simulink model "Pendulo_Adaptativo"  (R2023b)
settings: Solver=ode45  StartTime=0.0  StopTime=82  MaxStep=0.02  RelTol=1e-3
model workspace (MAT data in the model file):
  longitud = Simulink.Parameter
  longitud.Value = 0.6
  longitud.DataType = 'auto'
  longitud.Complexity = 'real'
  longitud.Dimensions = [1 1]
libraries: slpidlib x5
settings Model: Creator=Usuario  LastModifiedBy=Usuario
settings SolverCC: DaesscMode=Fast  ZeroCrossAlgorithm=Adaptive  EnableFixedStepZeroCrossing=on
settings DebuggingCC: IgnoredZcDiagnostic=none

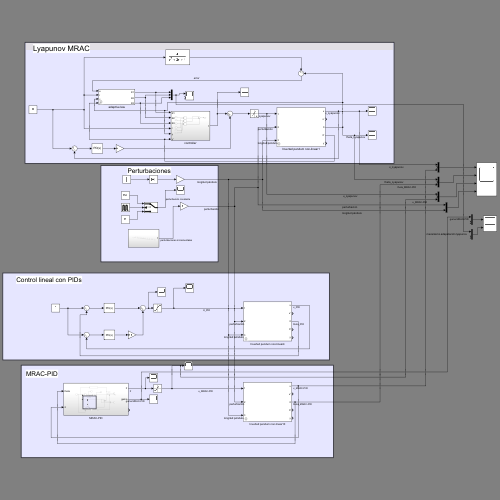
[thumbnail: Simulink's stored preview of the top-level diagram]
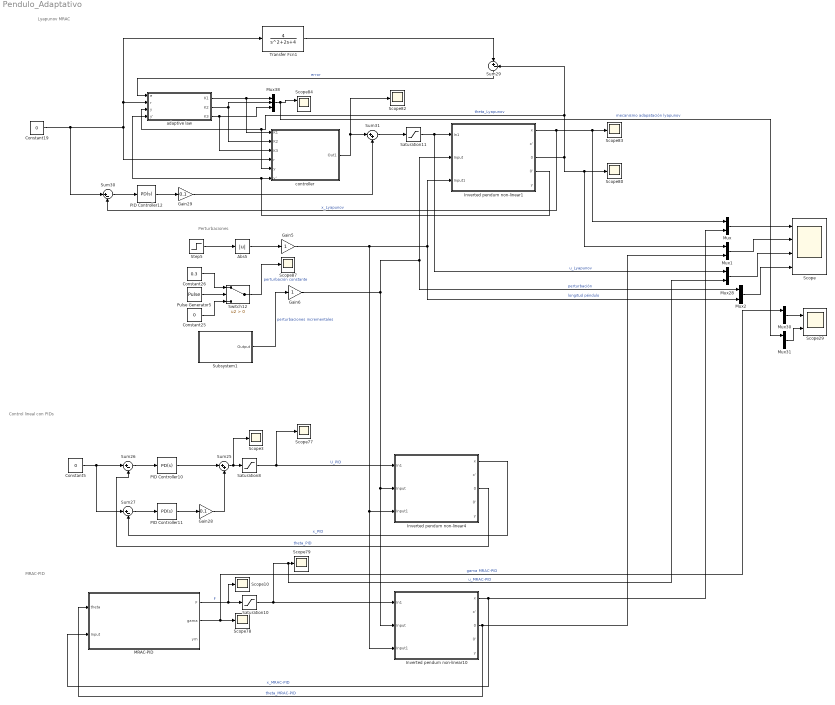
== system Pendulo_Adaptativo ==
  note: Lyapunov MRAC
  note: Perturbaciones
  note: Control lineal con PIDs
  note: MRAC-PID
  Abs5 : Abs  SaturateOnIntegerOverflow=off
  Constant19 : Constant  Value=0
  Constant25 : Constant  Value=0
  Constant26 : Constant  Value=0.3
  Constant5 : Constant  Value=0
  Gain28 : Gain  Gain=0.1
  Gain29 : Gain  Gain=0.1
  Gain5 : Gain
  Gain6 : Gain
  Inverted pendum non-linear1 : Subsystem  mask{M_=2, L=0.6, g=9.8, angulo=0.2, m=0.2}
      mask prompts: M_ "M"; angulo "angulo inicial"
  Inverted pendum non-linear10 : Subsystem  mask{M_=2, L=0.6, g=9.8, angulo=0.2, m=0.2}
      mask prompts: M_ "M"; angulo "angulo inicial"
  Inverted pendum non-linear4 : Subsystem  mask{M_=2, L=0.6, g=9.8, angulo=0.2, m=0.2}
      mask prompts: M_ "M"; angulo "angulo inicial"
  MRAC-PID : Subsystem
  Mux{,1,28,38} (4 alike) : Mux  Inputs=3
  Mux2 : Mux  Inputs=2
  Mux30 : Mux  Inputs=2
  Mux31 : Mux  Inputs=2
  PID Controller10 : slpidlib/PID Controller  Controller=PD  Form=Parallel  TimeDomain=Continuous-time  UseExternalTs=off  SampleTime=-1  IntegratorMethod=Forward Euler  FilterMethod=Forward Euler  ControllerParametersSource=internal  P=-30  I=0.01  UseKiTs=off  D=-10  N=100  UseFilter=on  TunerSelectOption=Transfer Function Based (PID Tuner App)  InitialConditionSource=internal  InitialConditionForIntegrator=0  InitialConditionForFilter=0  DifferentiatorICPrevScaledInput=0  ExternalReset=none  TrackingMode=off  Kt=1  LimitOutput=off  SatLimitsSource=internal  UpperSaturationLimit=inf  LowerSaturationLimit=-inf  LinearizeAsGain=on  AntiWindupMode=none  Kb=1  LimitIntegrator=off  UpperIntegratorSaturationLimit=inf  LowerIntegratorSaturationLimit=-inf  POutMin=[]  POutMax=[]  IOutMin=[]  IOutMax=[]  DOutMin=[]  DOutMax=[]  NOutMin=[]  NOutMax=[]  SumOutMin=[]  SumOutMax=[]  SaturationOutMin=[]  SaturationOutMax=[]  PParamMin=[]  PParamMax=[]  IParamMin=[]  IParamMax=[]  DParamMin=[]  DParamMax=[]  NParamMin=[]  NParamMax=[]  KbParamMin=[]  KbParamMax=[]  KtParamMin=[]  KtParamMax=[]  KbOutMin=[]  KbOutMax=[]  KtOutMin=[]  KtOutMax=[]  IntegratorOutMin=[]  IntegratorOutMax=[]  FilterOutMin=[]  FilterOutMax=[]  SumI1OutMin=[]  SumI1OutMax=[]  SumI2OutMin=[]  SumI2OutMax=[]  SumI3OutMin=[]  SumI3OutMax=[]  SumI4OutMin=[]  SumI4OutMax=[]  SumDOutMin=[]  SumDOutMax=[]  DifferentiatorOutMin=[]  DifferentiatorOutMax=[]  FilterDiffOutCoefMin=[]  FilterDiffOutCoefMax=[]  ReciprocalOutMin=[]  ReciprocalOutMax=[]  SumDenOutMin=[]  SumDenOutMax=[]  SumNumOutMin=[]  SumNumOutMax=[]  DivideOutMin=[]  DivideOutMax=[]  UdiffTsProdOutMin=[]  UdiffTsProdOutMax=[]  NTsProdOutMin=[]  NTsProdOutMax=[]  UintegralTsProdOutMin=[]  UintegralTsProdOutMax=[]  UngainTsProdOutMin=[]  UngainTsProdOutMax=[]  ClampingZeroOutDataTypeStr=Inherit: Inherit via back propagation  ClampingZeroOutMin=[]  ClampingZeroOutMax=[]  FilterDenConstantOutDataTypeStr=Inherit: Inherit via back propagation  FilterDenConstantOutMin=[]  FilterDenConstantOutMax=[]  PCopyOutDataTypeStr=Inherit: Inherit via back propagation  PCopyOutMin=[]  PCopyOutMax=[]  NCopyOutDataTypeStr=Inherit: Inherit via back propagation  NCopyOutMin=[]  NCopyOutMax=[]  IntegratorContinuousStateAttributes=''  IntegratorStateMustResolveToSignalObject=off  IntegratorRTWStateStorageClass=Auto  FilterContinuousStateAttributes=''  FilterStateMustResolveToSignalObject=off  FilterRTWStateStorageClass=Auto  ParallelPVariant=InternalParameters  IdealPVariant=Disabled  IVariant=Disabled  DVariant=InternalParameters  IntegratorVariant=Disabled  SatVariant=Disabled  AWVariant=Disabled  PCopyVariant=Disabled  TRVariant=Disabled  FdbkBlocksVariant=Forward  IdealPFdbkVariant=Disabled  SatFdbkVariant=Disabled  DerivativeFilterVariant=ContFilter  NVariant=InternalParameters  NCopyVariant=Disabled  FilterICVariant=InternalICsFilter  IntegratorICVariant=Disabled  ExternalResetVariant=Disabled  TRSumVariant=Passthrough  SumFdbkVariant=Disabled  SumVariant=Sum_PD  TsampFilterVariant=InternalTs  TsampNgainVariant=Passthrough  TsampIntegralVariant=Disabled_SignalSpec  ExternalSaturationOutDataTypeStr=Inherit: Same as second input
  PID Controller11 : slpidlib/PID Controller  Controller=PD  Form=Parallel  TimeDomain=Continuous-time  UseExternalTs=off  SampleTime=-1  IntegratorMethod=Forward Euler  FilterMethod=Forward Euler  ControllerParametersSource=internal  P=-3.5  I=0.01  UseKiTs=off  D=-10  N=10  UseFilter=on  TunerSelectOption=Transfer Function Based (PID Tuner App)  InitialConditionSource=internal  InitialConditionForIntegrator=0  InitialConditionForFilter=0  DifferentiatorICPrevScaledInput=0  ExternalReset=none  TrackingMode=off  Kt=1  LimitOutput=off  SatLimitsSource=internal  UpperSaturationLimit=inf  LowerSaturationLimit=-inf  LinearizeAsGain=on  AntiWindupMode=none  Kb=1  LimitIntegrator=off  UpperIntegratorSaturationLimit=inf  LowerIntegratorSaturationLimit=-inf  POutMin=[]  POutMax=[]  IOutMin=[]  IOutMax=[]  DOutMin=[]  DOutMax=[]  NOutMin=[]  NOutMax=[]  SumOutMin=[]  SumOutMax=[]  SaturationOutMin=[]  SaturationOutMax=[]  PParamMin=[]  PParamMax=[]  IParamMin=[]  IParamMax=[]  DParamMin=[]  DParamMax=[]  NParamMin=[]  NParamMax=[]  KbParamMin=[]  KbParamMax=[]  KtParamMin=[]  KtParamMax=[]  KbOutMin=[]  KbOutMax=[]  KtOutMin=[]  KtOutMax=[]  IntegratorOutMin=[]  IntegratorOutMax=[]  FilterOutMin=[]  FilterOutMax=[]  SumI1OutMin=[]  SumI1OutMax=[]  SumI2OutMin=[]  SumI2OutMax=[]  SumI3OutMin=[]  SumI3OutMax=[]  SumI4OutMin=[]  SumI4OutMax=[]  SumDOutMin=[]  SumDOutMax=[]  DifferentiatorOutMin=[]  DifferentiatorOutMax=[]  FilterDiffOutCoefMin=[]  FilterDiffOutCoefMax=[]  ReciprocalOutMin=[]  ReciprocalOutMax=[]  SumDenOutMin=[]  SumDenOutMax=[]  SumNumOutMin=[]  SumNumOutMax=[]  DivideOutMin=[]  DivideOutMax=[]  UdiffTsProdOutMin=[]  UdiffTsProdOutMax=[]  NTsProdOutMin=[]  NTsProdOutMax=[]  UintegralTsProdOutMin=[]  UintegralTsProdOutMax=[]  UngainTsProdOutMin=[]  UngainTsProdOutMax=[]  ClampingZeroOutDataTypeStr=Inherit: Inherit via back propagation  ClampingZeroOutMin=[]  ClampingZeroOutMax=[]  FilterDenConstantOutDataTypeStr=Inherit: Inherit via back propagation  FilterDenConstantOutMin=[]  FilterDenConstantOutMax=[]  PCopyOutDataTypeStr=Inherit: Inherit via back propagation  PCopyOutMin=[]  PCopyOutMax=[]  NCopyOutDataTypeStr=Inherit: Inherit via back propagation  NCopyOutMin=[]  NCopyOutMax=[]  IntegratorContinuousStateAttributes=''  IntegratorStateMustResolveToSignalObject=off  IntegratorRTWStateStorageClass=Auto  FilterContinuousStateAttributes=''  FilterStateMustResolveToSignalObject=off  FilterRTWStateStorageClass=Auto  ParallelPVariant=InternalParameters  IdealPVariant=Disabled  IVariant=Disabled  DVariant=InternalParameters  IntegratorVariant=Disabled  SatVariant=Disabled  AWVariant=Disabled  PCopyVariant=Disabled  TRVariant=Disabled  FdbkBlocksVariant=Forward  IdealPFdbkVariant=Disabled  SatFdbkVariant=Disabled  DerivativeFilterVariant=ContFilter  NVariant=InternalParameters  NCopyVariant=Disabled  FilterICVariant=InternalICsFilter  IntegratorICVariant=Disabled  ExternalResetVariant=Disabled  TRSumVariant=Passthrough  SumFdbkVariant=Disabled  SumVariant=Sum_PD  TsampFilterVariant=InternalTs  TsampNgainVariant=Passthrough  TsampIntegralVariant=Disabled_SignalSpec  ExternalSaturationOutDataTypeStr=Inherit: Same as second input
  PID Controller12 : slpidlib/PID Controller  Controller=PD  Form=Parallel  TimeDomain=Continuous-time  UseExternalTs=off  SampleTime=-1  IntegratorMethod=Forward Euler  FilterMethod=Forward Euler  ControllerParametersSource=internal  P=-3.5  I=0.01  UseKiTs=off  D=-10  N=10  UseFilter=on  TunerSelectOption=Transfer Function Based (PID Tuner App)  InitialConditionSource=internal  InitialConditionForIntegrator=0  InitialConditionForFilter=0  DifferentiatorICPrevScaledInput=0  ExternalReset=none  TrackingMode=off  Kt=1  LimitOutput=off  SatLimitsSource=internal  UpperSaturationLimit=inf  LowerSaturationLimit=-inf  LinearizeAsGain=on  AntiWindupMode=none  Kb=1  LimitIntegrator=off  UpperIntegratorSaturationLimit=inf  LowerIntegratorSaturationLimit=-inf  POutMin=[]  POutMax=[]  IOutMin=[]  IOutMax=[]  DOutMin=[]  DOutMax=[]  NOutMin=[]  NOutMax=[]  SumOutMin=[]  SumOutMax=[]  SaturationOutMin=[]  SaturationOutMax=[]  PParamMin=[]  PParamMax=[]  IParamMin=[]  IParamMax=[]  DParamMin=[]  DParamMax=[]  NParamMin=[]  NParamMax=[]  KbParamMin=[]  KbParamMax=[]  KtParamMin=[]  KtParamMax=[]  KbOutMin=[]  KbOutMax=[]  KtOutMin=[]  KtOutMax=[]  IntegratorOutMin=[]  IntegratorOutMax=[]  FilterOutMin=[]  FilterOutMax=[]  SumI1OutMin=[]  SumI1OutMax=[]  SumI2OutMin=[]  SumI2OutMax=[]  SumI3OutMin=[]  SumI3OutMax=[]  SumI4OutMin=[]  SumI4OutMax=[]  SumDOutMin=[]  SumDOutMax=[]  DifferentiatorOutMin=[]  DifferentiatorOutMax=[]  FilterDiffOutCoefMin=[]  FilterDiffOutCoefMax=[]  ReciprocalOutMin=[]  ReciprocalOutMax=[]  SumDenOutMin=[]  SumDenOutMax=[]  SumNumOutMin=[]  SumNumOutMax=[]  DivideOutMin=[]  DivideOutMax=[]  UdiffTsProdOutMin=[]  UdiffTsProdOutMax=[]  NTsProdOutMin=[]  NTsProdOutMax=[]  UintegralTsProdOutMin=[]  UintegralTsProdOutMax=[]  UngainTsProdOutMin=[]  UngainTsProdOutMax=[]  ClampingZeroOutDataTypeStr=Inherit: Inherit via back propagation  ClampingZeroOutMin=[]  ClampingZeroOutMax=[]  FilterDenConstantOutDataTypeStr=Inherit: Inherit via back propagation  FilterDenConstantOutMin=[]  FilterDenConstantOutMax=[]  PCopyOutDataTypeStr=Inherit: Inherit via back propagation  PCopyOutMin=[]  PCopyOutMax=[]  NCopyOutDataTypeStr=Inherit: Inherit via back propagation  NCopyOutMin=[]  NCopyOutMax=[]  IntegratorContinuousStateAttributes=''  IntegratorStateMustResolveToSignalObject=off  IntegratorRTWStateStorageClass=Auto  FilterContinuousStateAttributes=''  FilterStateMustResolveToSignalObject=off  FilterRTWStateStorageClass=Auto  ParallelPVariant=InternalParameters  IdealPVariant=Disabled  IVariant=Disabled  DVariant=InternalParameters  IntegratorVariant=Disabled  SatVariant=Disabled  AWVariant=Disabled  PCopyVariant=Disabled  TRVariant=Disabled  FdbkBlocksVariant=Forward  IdealPFdbkVariant=Disabled  SatFdbkVariant=Disabled  DerivativeFilterVariant=ContFilter  NVariant=InternalParameters  NCopyVariant=Disabled  FilterICVariant=InternalICsFilter  IntegratorICVariant=Disabled  ExternalResetVariant=Disabled  TRSumVariant=Passthrough  SumFdbkVariant=Disabled  SumVariant=Sum_PD  TsampFilterVariant=InternalTs  TsampNgainVariant=Passthrough  TsampIntegralVariant=Disabled_SignalSpec  ExternalSaturationOutDataTypeStr=Inherit: Same as second input
  Pulse Generator5 : DiscretePulseGenerator  PulseType=Time based  Period=10  PhaseDelay=10
  Saturation10 : Saturate  UpperLimit=10  LowerLimit=-10
  Saturation11 : Saturate  UpperLimit=10  LowerLimit=-10
  Saturation8 : Saturate  UpperLimit=10  LowerLimit=-10
  Scope : Scope  NumInputPorts=4
  Scope{3,10,77..80,82..83,87} (9 alike) : Scope
  Scope29 : Scope  NumInputPorts=2
  Scope84 : Scope  NumInputPorts=2
  Step5 : Step  Time=30.5  Before=0.6  After=2  SampleTime=0
  Subsystem1 : Subsystem
  Sum25 : Sum  Inputs=|++
  Sum{26..27,29..30} (4 alike) : Sum  Inputs=|+-
  Sum31 : Sum  Inputs=|++
  Switch12 : Switch  Criteria=u2 > Threshold  SaturateOnIntegerOverflow=off  InputSameDT=off
  Transfer Fcn1 : TransferFcn  Numerator=[4]  Denominator=[1 2 4]
  adaptive law : Subsystem  mask{p12=1/8, p22=5/16, gama1=-100, gama2=100, gama3=100, k1=-10, k2=-40, k3=-10}
  controller : Subsystem
  wires:
  PID Controller10/1 -> Sum25/1
  PID Controller11/1 -> Gain28/1
  Gain28/1 -> Sum25/2
  Sum26/1 -> PID Controller10/1
  Constant5/1 -> Sum27/1, Sum26/1
  Inverted pendum non-linear4/3(0) -> Sum26/2  "theta_PID"
  Inverted pendum non-linear4/1(x) -> Sum27/2  "x_PID"
  Sum27/1 -> PID Controller11/1
  Mux1/1 -> Scope/2
  Mux/1 -> Scope/1
  Mux28/1 -> Scope/3
  Sum25/1 -> Scope3/1, Saturation8/1
  Saturation8/1 -> Scope77/1, Inverted pendum non-linear4/1(In1)  "U_PID"
  Saturation10/1 -> Mux28/3, Scope79/1, Inverted pendum non-linear10/1(In1)  "u_MRAC-PID"
  MRAC-PID/1(F) -> Scope10/1, Saturation10/1  "F"
  MRAC-PID/2(gama) -> Mux30/1, Scope78/1  "gama MRAC-PID"
  Inverted pendum non-linear10/1(x) -> Mux/3, MRAC-PID/2(Input)  "x_MRAC-PID"
  Inverted pendum non-linear10/3(0) -> Mux1/3, MRAC-PID/1(theta)  "theta_MRAC-PID"
  adaptive law/2(K2) -> Mux38/2, controller/2(K2)
  adaptive law/3(K3) -> controller/3(K3), Mux38/3
  Constant19/1 -> controller/4(r), Transfer Fcn1/1, adaptive law/2(r), Sum30/1
  controller/1(Out1) -> Sum31/1, Scope82/1
  Transfer Fcn1/1 -> Sum29/1
  Inverted pendum non-linear1/3(0) -> Sum29/2, adaptive law/3(y), controller/5(y), Mux1/1, Scope80/1  "theta_Lyapunov"
  Sum29/1 -> adaptive law/1(e)  "error"
  Inverted pendum non-linear1/4(0') -> adaptive law/4(y'), controller/6(y')
  Inverted pendum non-linear1/1(x) -> Mux/1, Scope83/1, Sum30/2  "x_Lyapunov"
  adaptive law/1(K1) -> Mux38/1, controller/1(K1)
  Mux38/1 -> Mux31/1, Scope84/1  "mecanismo adapatación lyapunov"
  Switch12/1 -> Scope87/1  "perturbación constante"
  Constant26/1 -> Switch12/1
  Constant25/1 -> Switch12/3
  Pulse Generator5/1 -> Switch12/2
  Step5/1 -> Abs5/1
  PID Controller12/1 -> Gain29/1
  Sum30/1 -> PID Controller12/1
  Sum31/1 -> Saturation11/1
  Gain29/1 -> Sum31/2
  Saturation11/1 -> Mux28/1, Inverted pendum non-linear1/1(In1)  "u_Lyapunov"
  Mux2/1 -> Scope/4
  Gain5/1 -> Inverted pendum non-linear4/3(Input1), Inverted pendum non-linear10/3(Input1), Mux2/2, Inverted pendum non-linear1/3(Input1)  "longitud péndulo"
  Gain6/1 -> Mux2/1, Inverted pendum non-linear1/2(Input), Inverted pendum non-linear4/2(Input), Inverted pendum non-linear10/2(Input)  "perturbación"
  Abs5/1 -> Gain5/1
  Mux30/1 -> Scope29/1
  Mux31/1 -> Scope29/2
  Subsystem1/1(Output) -> Gain6/1  "perturbaciones incrementales"

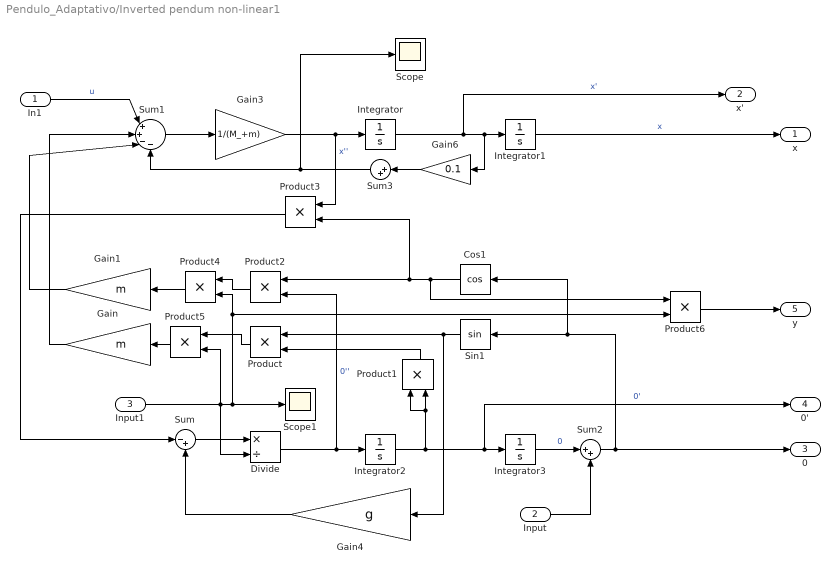
== system Pendulo_Adaptativo/Inverted pendum non-linear1 ==
  In1 : Inport
  Input : Inport  Port=2
  Input1 : Inport  Port=3
  Cos1 : Trigonometry  Operator=cos
  Divide : Product  Inputs=*/
  Gain : Gain  Gain=m
  Gain1 : Gain  Gain=m
  Gain3 : Gain  Gain=1/(M_+m)
  Gain4 : Gain  Gain=g
  Gain6 : Gain  Gain=0.1
  Integrator : Integrator
  Integrator1 : Integrator
  Integrator2 : Integrator
  Integrator3 : Integrator  InitialCondition=angulo
  Product{,1..6} (7 alike) : Product
  Scope : Scope
  Scope1 : Scope
  Sin1 : Trigonometry
  Sum : Sum  Inputs=|-+
  Sum1 : Sum  Inputs=|++--
  Sum2 : Sum  Inputs=|++
  Sum3 : Sum  Inputs=|++
  x : Outport
  x' : Outport  Port=2
  0 : Outport  Port=3
  0' : Outport  Port=4
  y : Outport  Port=5
  wires:
  Integrator2/1 -> Product1/1, Product1/2, Integrator3/1, 0'/1  "0'"
  Integrator1/1 -> x/1  "x"
  Integrator3/1 -> Sum2/1  "0"
  Cos1/1 -> Product6/1, Product3/2, Product2/1
  Sin1/1 -> Gain4/1, Product/1
  Product1/1 -> Product/2
  Gain/1 -> Sum1/2
  Gain1/1 -> Sum1/3
  Product3/1 -> Sum/1
  Gain4/1 -> Sum/2
  Sum1/1 -> Gain3/1
  Gain3/1 -> Product3/1, Integrator/1  "x''"
  In1/1 -> Sum1/1  "u"
  Sum/1 -> Divide/1
  Divide/1 -> Product2/2, Integrator2/1  "0''"
  Product6/1 -> y/1
  Sum2/1 -> Cos1/1, Sin1/1, 0/1
  Input/1 -> Sum2/2
  Product4/1 -> Gain1/1
  Product2/1 -> Product4/1
  Input1/1 -> Product5/2, Scope1/1, Product6/2, Product4/2, Divide/2
  Product5/1 -> Gain/1
  Product/1 -> Product5/1
  Sum3/1 -> Scope/1, Sum1/4
  Gain6/1 -> Sum3/1
  Integrator/1 -> Gain6/1, Integrator1/1, x'/1  "x'"

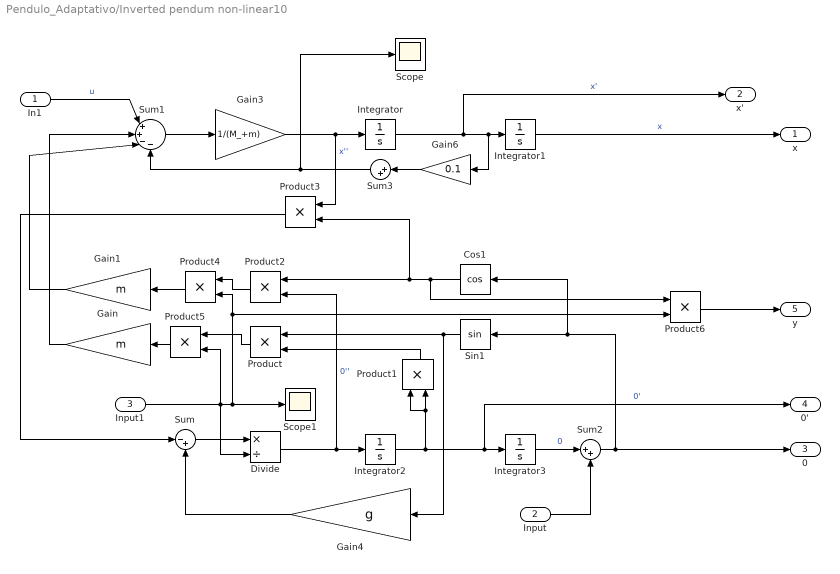
== system Pendulo_Adaptativo/Inverted pendum non-linear10 ==
  In1 : Inport
  Input : Inport  Port=2
  Input1 : Inport  Port=3
  Cos1 : Trigonometry  Operator=cos
  Divide : Product  Inputs=*/
  Gain : Gain  Gain=m
  Gain1 : Gain  Gain=m
  Gain3 : Gain  Gain=1/(M_+m)
  Gain4 : Gain  Gain=g
  Gain6 : Gain  Gain=0.1
  Integrator : Integrator
  Integrator1 : Integrator
  Integrator2 : Integrator
  Integrator3 : Integrator  InitialCondition=angulo
  Product{,1..6} (7 alike) : Product
  Scope : Scope
  Scope1 : Scope
  Sin1 : Trigonometry
  Sum : Sum  Inputs=|-+
  Sum1 : Sum  Inputs=|++--
  Sum2 : Sum  Inputs=|++
  Sum3 : Sum  Inputs=|++
  x : Outport
  x' : Outport  Port=2
  0 : Outport  Port=3
  0' : Outport  Port=4
  y : Outport  Port=5
  wires:
  Integrator/1 -> Gain6/1, Integrator1/1, x'/1  "x'"
  Integrator2/1 -> Product1/1, Product1/2, Integrator3/1, 0'/1  "0'"
  Integrator1/1 -> x/1  "x"
  Integrator3/1 -> Sum2/1  "0"
  Cos1/1 -> Product6/1, Product3/2, Product2/1
  Sin1/1 -> Gain4/1, Product/1
  Product1/1 -> Product/2
  Gain/1 -> Sum1/2
  Gain1/1 -> Sum1/3
  Product3/1 -> Sum/1
  Gain4/1 -> Sum/2
  Sum1/1 -> Gain3/1
  Gain3/1 -> Product3/1, Integrator/1  "x''"
  In1/1 -> Sum1/1  "u"
  Sum/1 -> Divide/1
  Divide/1 -> Product2/2, Integrator2/1  "0''"
  Product6/1 -> y/1
  Sum2/1 -> Cos1/1, Sin1/1, 0/1
  Input/1 -> Sum2/2
  Product4/1 -> Gain1/1
  Product2/1 -> Product4/1
  Input1/1 -> Product5/2, Scope1/1, Product6/2, Product4/2, Divide/2
  Product5/1 -> Gain/1
  Product/1 -> Product5/1
  Sum3/1 -> Scope/1, Sum1/4
  Gain6/1 -> Sum3/1

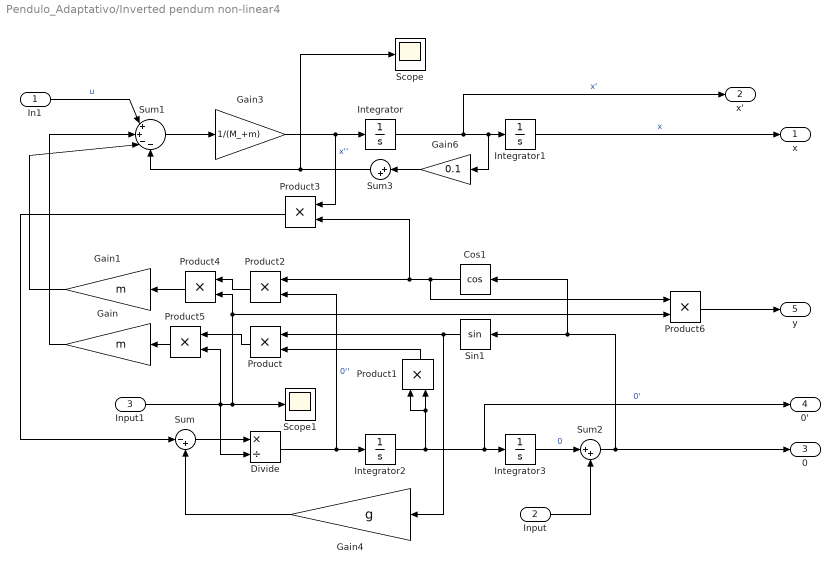
== system Pendulo_Adaptativo/Inverted pendum non-linear4 ==
  In1 : Inport
  Input : Inport  Port=2
  Input1 : Inport  Port=3
  Cos1 : Trigonometry  Operator=cos
  Divide : Product  Inputs=*/
  Gain : Gain  Gain=m
  Gain1 : Gain  Gain=m
  Gain3 : Gain  Gain=1/(M_+m)
  Gain4 : Gain  Gain=g
  Gain6 : Gain  Gain=0.1
  Integrator : Integrator
  Integrator1 : Integrator
  Integrator2 : Integrator
  Integrator3 : Integrator  InitialCondition=angulo
  Product{,1..6} (7 alike) : Product
  Scope : Scope
  Scope1 : Scope
  Sin1 : Trigonometry
  Sum : Sum  Inputs=|-+
  Sum1 : Sum  Inputs=|++--
  Sum2 : Sum  Inputs=|++
  Sum3 : Sum  Inputs=|++
  x : Outport
  x' : Outport  Port=2
  0 : Outport  Port=3
  0' : Outport  Port=4
  y : Outport  Port=5
  wires:
  Integrator2/1 -> Product1/1, Product1/2, Integrator3/1, 0'/1  "0'"
  Integrator1/1 -> x/1  "x"
  Integrator3/1 -> Sum2/1  "0"
  Cos1/1 -> Product6/1, Product3/2, Product2/1
  Sin1/1 -> Gain4/1, Product/1
  Product1/1 -> Product/2
  Gain/1 -> Sum1/2
  Gain1/1 -> Sum1/3
  Product3/1 -> Sum/1
  Gain4/1 -> Sum/2
  Sum1/1 -> Gain3/1
  Gain3/1 -> Product3/1, Integrator/1  "x''"
  In1/1 -> Sum1/1  "u"
  Sum/1 -> Divide/1
  Divide/1 -> Product2/2, Integrator2/1  "0''"
  Product6/1 -> y/1
  Sum2/1 -> Cos1/1, Sin1/1, 0/1
  Input/1 -> Sum2/2
  Product4/1 -> Gain1/1
  Product2/1 -> Product4/1
  Input1/1 -> Product5/2, Scope1/1, Product6/2, Product4/2, Divide/2
  Product5/1 -> Gain/1
  Product/1 -> Product5/1
  Sum3/1 -> Scope/1, Sum1/4
  Gain6/1 -> Sum3/1
  Integrator/1 -> Gain6/1, Integrator1/1, x'/1  "x'"

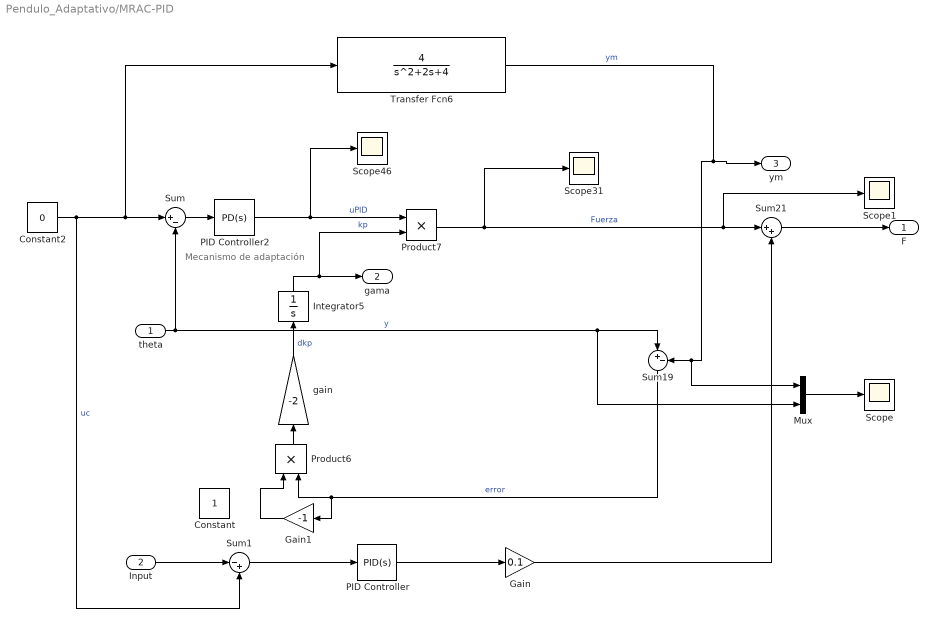
== system Pendulo_Adaptativo/MRAC-PID ==
  note: Mecanismo de adaptación
  theta : Inport
  Input : Inport  Port=2
  Constant : Constant
  Constant2 : Constant  Value=0
  Gain : Gain  Gain=0.1
  Gain1 : Gain  Gain=-1
  Integrator5 : Integrator  InitialCondition=2
  Mux : Mux  Inputs=2
  PID Controller : slpidlib/PID Controller  Controller=PID  Form=Parallel  TimeDomain=Continuous-time  UseExternalTs=off  SampleTime=-1  IntegratorMethod=Forward Euler  FilterMethod=Forward Euler  ControllerParametersSource=internal  P=-3.5  I=0  UseKiTs=off  D=-10  N=10  UseFilter=on  TunerSelectOption=Transfer Function Based (PID Tuner App)  InitialConditionSource=internal  InitialConditionForIntegrator=0  InitialConditionForFilter=0  DifferentiatorICPrevScaledInput=0  ExternalReset=none  TrackingMode=off  Kt=1  LimitOutput=off  SatLimitsSource=internal  UpperSaturationLimit=inf  LowerSaturationLimit=-inf  LinearizeAsGain=on  AntiWindupMode=none  Kb=1  LimitIntegrator=off  UpperIntegratorSaturationLimit=inf  LowerIntegratorSaturationLimit=-inf  POutMin=[]  POutMax=[]  IOutMin=[]  IOutMax=[]  DOutMin=[]  DOutMax=[]  NOutMin=[]  NOutMax=[]  SumOutMin=[]  SumOutMax=[]  SaturationOutMin=[]  SaturationOutMax=[]  PParamMin=[]  PParamMax=[]  IParamMin=[]  IParamMax=[]  DParamMin=[]  DParamMax=[]  NParamMin=[]  NParamMax=[]  KbParamMin=[]  KbParamMax=[]  KtParamMin=[]  KtParamMax=[]  KbOutMin=[]  KbOutMax=[]  KtOutMin=[]  KtOutMax=[]  IntegratorOutMin=[]  IntegratorOutMax=[]  FilterOutMin=[]  FilterOutMax=[]  SumI1OutMin=[]  SumI1OutMax=[]  SumI2OutMin=[]  SumI2OutMax=[]  SumI3OutMin=[]  SumI3OutMax=[]  SumI4OutMin=[]  SumI4OutMax=[]  SumDOutMin=[]  SumDOutMax=[]  DifferentiatorOutMin=[]  DifferentiatorOutMax=[]  FilterDiffOutCoefMin=[]  FilterDiffOutCoefMax=[]  ReciprocalOutMin=[]  ReciprocalOutMax=[]  SumDenOutMin=[]  SumDenOutMax=[]  SumNumOutMin=[]  SumNumOutMax=[]  DivideOutMin=[]  DivideOutMax=[]  UdiffTsProdOutMin=[]  UdiffTsProdOutMax=[]  NTsProdOutMin=[]  NTsProdOutMax=[]  UintegralTsProdOutMin=[]  UintegralTsProdOutMax=[]  UngainTsProdOutMin=[]  UngainTsProdOutMax=[]  ClampingZeroOutDataTypeStr=Inherit: Inherit via back propagation  ClampingZeroOutMin=[]  ClampingZeroOutMax=[]  FilterDenConstantOutDataTypeStr=Inherit: Inherit via back propagation  FilterDenConstantOutMin=[]  FilterDenConstantOutMax=[]  PCopyOutDataTypeStr=Inherit: Inherit via back propagation  PCopyOutMin=[]  PCopyOutMax=[]  NCopyOutDataTypeStr=Inherit: Inherit via back propagation  NCopyOutMin=[]  NCopyOutMax=[]  IntegratorContinuousStateAttributes=''  IntegratorStateMustResolveToSignalObject=off  IntegratorRTWStateStorageClass=Auto  FilterContinuousStateAttributes=''  FilterStateMustResolveToSignalObject=off  FilterRTWStateStorageClass=Auto  ParallelPVariant=InternalParameters  IdealPVariant=Disabled  IVariant=InternalParameters  DVariant=InternalParameters  IntegratorVariant=Continuous  SatVariant=Disabled  AWVariant=Passthrough  PCopyVariant=Disabled  TRVariant=Disabled  FdbkBlocksVariant=Forward  IdealPFdbkVariant=Disabled  SatFdbkVariant=Disabled  DerivativeFilterVariant=ContFilter  NVariant=InternalParameters  NCopyVariant=Disabled  FilterICVariant=InternalICsFilter  IntegratorICVariant=InternalICs  ExternalResetVariant=Disabled  TRSumVariant=Passthrough  SumFdbkVariant=Disabled  SumVariant=Sum_PID  TsampFilterVariant=InternalTs  TsampNgainVariant=Passthrough  TsampIntegralVariant=Disabled_SignalSpec  ExternalSaturationOutDataTypeStr=Inherit: Same as second input
  PID Controller2 : slpidlib/PID Controller  Controller=PD  Form=Parallel  TimeDomain=Continuous-time  UseExternalTs=off  SampleTime=-1  IntegratorMethod=Forward Euler  FilterMethod=Forward Euler  ControllerParametersSource=internal  P=-30  I=0.01  UseKiTs=off  D=-10  N=100  UseFilter=on  TunerSelectOption=Transfer Function Based (PID Tuner App)  InitialConditionSource=internal  InitialConditionForIntegrator=0  InitialConditionForFilter=0  DifferentiatorICPrevScaledInput=0  ExternalReset=none  TrackingMode=off  Kt=1  LimitOutput=off  SatLimitsSource=internal  UpperSaturationLimit=inf  LowerSaturationLimit=-inf  LinearizeAsGain=on  AntiWindupMode=none  Kb=1  LimitIntegrator=off  UpperIntegratorSaturationLimit=inf  LowerIntegratorSaturationLimit=-inf  POutMin=[]  POutMax=[]  IOutMin=[]  IOutMax=[]  DOutMin=[]  DOutMax=[]  NOutMin=[]  NOutMax=[]  SumOutMin=[]  SumOutMax=[]  SaturationOutMin=[]  SaturationOutMax=[]  PParamMin=[]  PParamMax=[]  IParamMin=[]  IParamMax=[]  DParamMin=[]  DParamMax=[]  NParamMin=[]  NParamMax=[]  KbParamMin=[]  KbParamMax=[]  KtParamMin=[]  KtParamMax=[]  KbOutMin=[]  KbOutMax=[]  KtOutMin=[]  KtOutMax=[]  IntegratorOutMin=[]  IntegratorOutMax=[]  FilterOutMin=[]  FilterOutMax=[]  SumI1OutMin=[]  SumI1OutMax=[]  SumI2OutMin=[]  SumI2OutMax=[]  SumI3OutMin=[]  SumI3OutMax=[]  SumI4OutMin=[]  SumI4OutMax=[]  SumDOutMin=[]  SumDOutMax=[]  DifferentiatorOutMin=[]  DifferentiatorOutMax=[]  FilterDiffOutCoefMin=[]  FilterDiffOutCoefMax=[]  ReciprocalOutMin=[]  ReciprocalOutMax=[]  SumDenOutMin=[]  SumDenOutMax=[]  SumNumOutMin=[]  SumNumOutMax=[]  DivideOutMin=[]  DivideOutMax=[]  UdiffTsProdOutMin=[]  UdiffTsProdOutMax=[]  NTsProdOutMin=[]  NTsProdOutMax=[]  UintegralTsProdOutMin=[]  UintegralTsProdOutMax=[]  UngainTsProdOutMin=[]  UngainTsProdOutMax=[]  ClampingZeroOutDataTypeStr=Inherit: Inherit via back propagation  ClampingZeroOutMin=[]  ClampingZeroOutMax=[]  FilterDenConstantOutDataTypeStr=Inherit: Inherit via back propagation  FilterDenConstantOutMin=[]  FilterDenConstantOutMax=[]  PCopyOutDataTypeStr=Inherit: Inherit via back propagation  PCopyOutMin=[]  PCopyOutMax=[]  NCopyOutDataTypeStr=Inherit: Inherit via back propagation  NCopyOutMin=[]  NCopyOutMax=[]  IntegratorContinuousStateAttributes=''  IntegratorStateMustResolveToSignalObject=off  IntegratorRTWStateStorageClass=Auto  FilterContinuousStateAttributes=''  FilterStateMustResolveToSignalObject=off  FilterRTWStateStorageClass=Auto  ParallelPVariant=InternalParameters  IdealPVariant=Disabled  IVariant=Disabled  DVariant=InternalParameters  IntegratorVariant=Disabled  SatVariant=Disabled  AWVariant=Disabled  PCopyVariant=Disabled  TRVariant=Disabled  FdbkBlocksVariant=Forward  IdealPFdbkVariant=Disabled  SatFdbkVariant=Disabled  DerivativeFilterVariant=ContFilter  NVariant=InternalParameters  NCopyVariant=Disabled  FilterICVariant=InternalICsFilter  IntegratorICVariant=Disabled  ExternalResetVariant=Disabled  TRSumVariant=Passthrough  SumFdbkVariant=Disabled  SumVariant=Sum_PD  TsampFilterVariant=InternalTs  TsampNgainVariant=Passthrough  TsampIntegralVariant=Disabled_SignalSpec  ExternalSaturationOutDataTypeStr=Inherit: Same as second input
  Product6 : Product
  Product7 : Product
  Scope{,1,31,46} (4 alike) : Scope
  Sum : Sum  Inputs=|+-
  Sum1 : Sum  Inputs=|-+
  Sum19 : Sum  Inputs=|+-
  Sum21 : Sum  Inputs=|++
  Transfer Fcn6 : TransferFcn  Numerator=[4]  Denominator=[1 2 4]
  gain : Gain  Gain=-2
  F : Outport
  gama : Outport  Port=2
  ym : Outport  Port=3
  wires:
  Sum19/1 -> Gain1/1, Product6/2  "error"
  Constant2/1 -> Transfer Fcn6/1, Sum/1, Sum1/2  "uc"
  gain/1 -> Integrator5/1  "dkp"
  Sum21/1 -> F/1
  Sum/1 -> PID Controller2/1
  Integrator5/1 -> Product7/2, gama/1  "kp"
  PID Controller2/1 -> Product7/1, Scope46/1  "uPID"
  Product6/1 -> gain/1
  Transfer Fcn6/1 -> Mux/1, Sum19/2, ym/1  "ym"
  Product7/1 -> Sum21/1, Scope1/1, Scope31/1  "Fuerza"
  theta/1 -> Sum/2, Mux/2, Sum19/1  "y"
  Input/1 -> Sum1/1
  Sum1/1 -> PID Controller/1
  PID Controller/1 -> Gain/1
  Gain/1 -> Sum21/2
  Mux/1 -> Scope/1
  Gain1/1 -> Product6/1

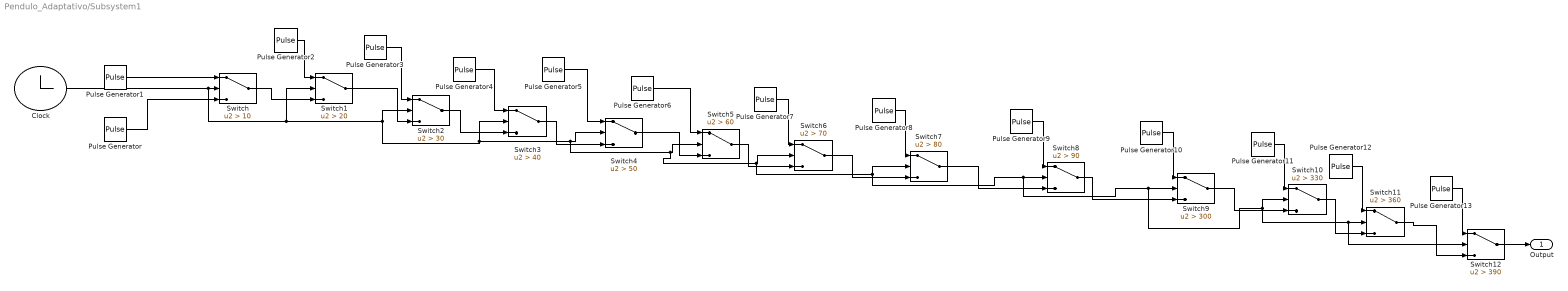
== system Pendulo_Adaptativo/Subsystem1 ==
  Clock : Clock
  Pulse Generator : DiscretePulseGenerator  PulseType=Time based  Amplitude=0  Period=30  PulseWidth=50
  Pulse Generator1 : DiscretePulseGenerator  PulseType=Time based  Amplitude=0.1  Period=30  PhaseDelay=11
  Pulse Generator10 : DiscretePulseGenerator  PulseType=Time based  Period=30  PhaseDelay=101
  Pulse Generator11 : DiscretePulseGenerator  PulseType=Time based  Amplitude=2.3  Period=30  PulseWidth=50  PhaseDelay=330
  Pulse Generator12 : DiscretePulseGenerator  PulseType=Time based  Amplitude=2.5  Period=30  PulseWidth=50  PhaseDelay=360
  Pulse Generator13 : DiscretePulseGenerator  PulseType=Time based  Amplitude=2.7  Period=30  PulseWidth=50  PhaseDelay=390
  Pulse Generator2 : DiscretePulseGenerator  PulseType=Time based  Amplitude=0.2  Period=30  PhaseDelay=21
  Pulse Generator3 : DiscretePulseGenerator  PulseType=Time based  Amplitude=0.3  Period=30  PhaseDelay=31
  Pulse Generator4 : DiscretePulseGenerator  PulseType=Time based  Amplitude=0.4  Period=30  PhaseDelay=41
  Pulse Generator5 : DiscretePulseGenerator  PulseType=Time based  Amplitude=0.5  Period=30  PhaseDelay=51
  Pulse Generator6 : DiscretePulseGenerator  PulseType=Time based  Amplitude=0.6  Period=30  PhaseDelay=61
  Pulse Generator7 : DiscretePulseGenerator  PulseType=Time based  Amplitude=0.7  Period=30  PhaseDelay=71
  Pulse Generator8 : DiscretePulseGenerator  PulseType=Time based  Amplitude=0.8  Period=30  PhaseDelay=81
  Pulse Generator9 : DiscretePulseGenerator  PulseType=Time based  Amplitude=0.9  Period=30  PhaseDelay=91
  Switch : Switch  Criteria=u2 > Threshold  Threshold=10  SaturateOnIntegerOverflow=off  InputSameDT=off
  Switch1 : Switch  Criteria=u2 > Threshold  Threshold=20  SaturateOnIntegerOverflow=off  InputSameDT=off
  Switch10 : Switch  Criteria=u2 > Threshold  Threshold=330  SaturateOnIntegerOverflow=off  InputSameDT=off
  Switch11 : Switch  Criteria=u2 > Threshold  Threshold=360  SaturateOnIntegerOverflow=off  InputSameDT=off
  Switch12 : Switch  Criteria=u2 > Threshold  Threshold=390  SaturateOnIntegerOverflow=off  InputSameDT=off
  Switch2 : Switch  Criteria=u2 > Threshold  Threshold=30  SaturateOnIntegerOverflow=off  InputSameDT=off
  Switch3 : Switch  Criteria=u2 > Threshold  Threshold=40  SaturateOnIntegerOverflow=off  InputSameDT=off
  Switch4 : Switch  Criteria=u2 > Threshold  Threshold=50  SaturateOnIntegerOverflow=off  InputSameDT=off
  Switch5 : Switch  Criteria=u2 > Threshold  Threshold=60  SaturateOnIntegerOverflow=off  InputSameDT=off
  Switch6 : Switch  Criteria=u2 > Threshold  Threshold=70  SaturateOnIntegerOverflow=off  InputSameDT=off
  Switch7 : Switch  Criteria=u2 > Threshold  Threshold=80  SaturateOnIntegerOverflow=off  InputSameDT=off
  Switch8 : Switch  Criteria=u2 > Threshold  Threshold=90  SaturateOnIntegerOverflow=off  InputSameDT=off
  Switch9 : Switch  Criteria=u2 > Threshold  Threshold=300  SaturateOnIntegerOverflow=off  InputSameDT=off
  Output : Outport
  wires:
  Pulse Generator1/1 -> Switch/1
  Pulse Generator/1 -> Switch/3
  Switch/1 -> Switch1/3
  Switch1/1 -> Switch2/3
  Pulse Generator3/1 -> Switch2/1
  Pulse Generator2/1 -> Switch1/1
  Pulse Generator4/1 -> Switch3/1
  Switch2/1 -> Switch3/3
  Pulse Generator5/1 -> Switch4/1
  Switch3/1 -> Switch4/3
  Pulse Generator6/1 -> Switch5/1
  Switch4/1 -> Switch5/3
  Pulse Generator7/1 -> Switch6/1
  Switch5/1 -> Switch6/3
  Pulse Generator8/1 -> Switch7/1
  Pulse Generator9/1 -> Switch8/1
  Switch7/1 -> Switch8/3
  Switch8/1 -> Switch9/3
  Pulse Generator10/1 -> Switch9/1
  Switch6/1 -> Switch7/3
  Pulse Generator11/1 -> Switch10/1
  Switch9/1 -> Switch10/3
  Switch10/1 -> Switch11/3
  Pulse Generator12/1 -> Switch11/1
  Pulse Generator13/1 -> Switch12/1
  Switch12/1 -> Output/1
  Clock/1 -> Switch3/2, Switch7/2, Switch8/2, Switch10/2, Switch12/2, Switch11/2, Switch9/2, Switch6/2, Switch5/2, Switch4/2, Switch2/2, Switch1/2, Switch/2
  Switch11/1 -> Switch12/3

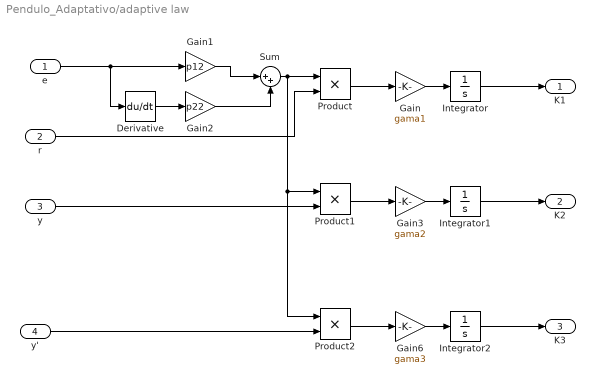
== system Pendulo_Adaptativo/adaptive law ==
  e : Inport
  r : Inport  Port=2
  y : Inport  Port=3
  y' : Inport  Port=4
  Derivative : Derivative
  Gain : Gain  Gain=gama1
  Gain1 : Gain  Gain=p12
  Gain2 : Gain  Gain=p22
  Gain3 : Gain  Gain=gama2
  Gain6 : Gain  Gain=gama3
  Integrator : Integrator  InitialCondition=k1
  Integrator1 : Integrator  InitialCondition=k2
  Integrator2 : Integrator  InitialCondition=k3
  Product : Product
  Product1 : Product
  Product2 : Product
  Sum : Sum  Inputs=|++
  K1 : Outport
  K2 : Outport  Port=2
  K3 : Outport  Port=3
  wires:
  Integrator/1 -> K1/1
  Gain/1 -> Integrator/1
  Derivative/1 -> Gain2/1
  Gain2/1 -> Sum/2
  Gain1/1 -> Sum/1
  Product/1 -> Gain/1
  r/1 -> Product/2
  Gain3/1 -> Integrator1/1
  Product1/1 -> Gain3/1
  e/1 -> Derivative/1, Gain1/1
  y/1 -> Product1/2
  Gain6/1 -> Integrator2/1
  Product2/1 -> Gain6/1
  Sum/1 -> Product/1, Product2/1, Product1/1
  y'/1 -> Product2/2
  Integrator2/1 -> K3/1
  Integrator1/1 -> K2/1

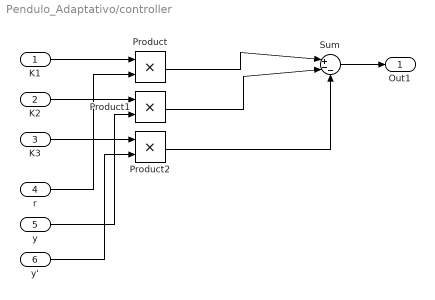
== system Pendulo_Adaptativo/controller ==
  K1 : Inport
  K2 : Inport  Port=2
  K3 : Inport  Port=3
  r : Inport  Port=4
  y : Inport  Port=5
  y' : Inport  Port=6
  Product : Product
  Product1 : Product
  Product2 : Product
  Sum : Sum  Inputs=|+--
  Out1 : Outport
  wires:
  Sum/1 -> Out1/1
  K1/1 -> Product/1
  Product/1 -> Sum/1
  r/1 -> Product/2
  K2/1 -> Product1/1
  K3/1 -> Product2/1
  y/1 -> Product1/2
  y'/1 -> Product2/2
  Product2/1 -> Sum/3
  Product1/1 -> Sum/2
